simulink model "Figure_2_2_TP_Telecom_modulation_demodulation_ASK2"  (R2020a)
settings: Solver=VariableStepAuto  StartTime=0.0  StopTime=10.0  RelTol=1e-3
libraries: simulink x2, dspsigops x2, dspsrcs4 x2, commrandsrc3 x1, dsparch4 x1, commsink2 x1, commfilt2 x1, commutil2 x1
settings Model: Creator=iba  LastModifiedBy=iba

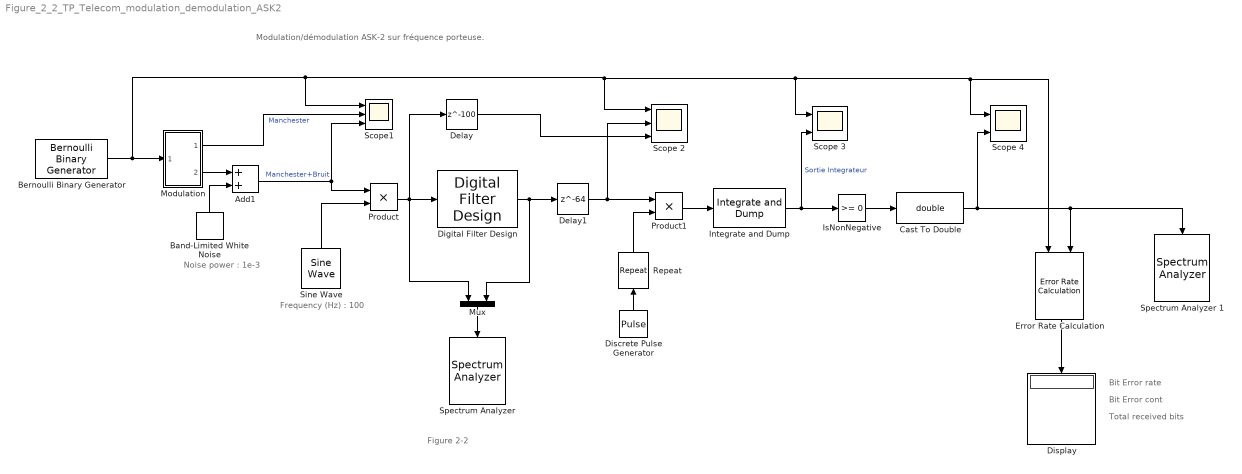
== system Figure_2_2_TP_Telecom_modulation_demodulation_ASK2 ==
  note: Figure 2-2
  note: Noise power : 1e-3
  note: Modulation/démodulation ASK-2 sur fréquence porteuse.
  note: Frequency (Hz) : 100
  note: Bit Error rate
  note: Bit Error cont
  note: Total received bits
  Add1 : Sum
  "Band-Limited White Noise " : simulink/Sources/Band-Limited White Noise  Cov=[1e-3]  Ts=1  seed=[1]
  "Bernoulli Binary Generator " : commrandsrc3/Bernoulli Binary Generator  ProbabilityOfZero=0.5  SeedSource=Parameter  Seed=25.  SampleTime=1  SamplesPerFrame=1  OutputDataType=double  SimulateUsing=Interpreted execution
  Cast To Double : DataTypeConversion  OutDataTypeStr=double
  "Delay " : Delay  DelayLength=100  InitialCondition=0
  "Delay1 " : Delay  DelayLength=64  InitialCondition=0
  "Digital Filter Design " : dsparch4/Digital Filter Design  mwdsp_browser_bugfix_var=off
  Discrete Pulse Generator : DiscretePulseGenerator  Period=10  PulseWidth=4
  "Display " : Display
  Error Rate Calculation : commsink2/Error Rate Calculation  N=1  st_delay=0  cp_mode=Entire frame  subframe=[]  PMode=Port  WsName=ErrorVec  RsMode2=off  stop=off  numErr=100  maxBits=1e6
  Integrate and Dump : commfilt2/Integrate and Dump  obssamples=2  offsetsamples=0  nodump=off  roundingMode=Floor  overflowMode=off
  IsNonNegative : simulink/Logic and Bit Operations/Compare To Zero  relop=>=  OutDataTypeStr=boolean
  Modulation : Subsystem
  Mux : Mux  Inputs=2
  "Product " : Product
  "Product1 " : Product
  Repeat : dspsigops/Repeat  N=50  RateOptions=Allow multirate processing  ic=0  mode=Unused parameter value
  Scope 2 : Scope  NumInputPorts=3
  Scope 3 : Scope  NumInputPorts=2
  Scope 4 : Scope  NumInputPorts=2
  "Scope1 " : Scope  NumInputPorts=3
  Sine Wave : dspsrcs4/Sine Wave  Amplitude=1  Frequency=100  Phase=0  SampleMode=Discrete  OutComplex=Real  CompMethod=Trigonometric fcn  TableSize=Speed  SampleTime=1  SamplesPerFrame=1  ResetState=Restart at time zero  OutputFrames=off  dataType=double  wordLen=16  udDataType=sfix(16)  fracBitsMode=Best precision  numFracBits=15  OutDataTypeStr=double  LastOutDataTypeStr=double
  "Spectrum Analyzer " : SpectrumAnalyzer
  Spectrum Analyzer 1 : SpectrumAnalyzer
  wires:
  "Bernoulli Binary Generator "/1 -> "Scope1 "/1, Error Rate Calculation/1, Scope 4/1, Scope 3/1, Scope 2/1, Modulation/1(IN1)
  Modulation/1(OUT1) -> "Scope1 "/2  "Manchester"
  Modulation/2(OUT2) -> Add1/1
  "Band-Limited White Noise "/1 -> Add1/2
  Add1/1 -> "Scope1 "/3, "Product "/1  "Manchester+Bruit"
  Sine Wave/1 -> "Product "/2
  "Product "/1 -> Mux/1, "Delay "/1, "Digital Filter Design "/1
  "Digital Filter Design "/1 -> "Delay1 "/1, Mux/2
  Mux/1 -> "Spectrum Analyzer "/1
  "Delay1 "/1 -> Scope 2/2, "Product1 "/1
  "Delay "/1 -> Scope 2/3
  "Product1 "/1 -> Integrate and Dump/1
  Repeat/1 -> "Product1 "/2
  Discrete Pulse Generator/1 -> Repeat/1
  Cast To Double/1 -> Scope 4/2, Spectrum Analyzer 1/1, Error Rate Calculation/2
  Integrate and Dump/1 -> Scope 3/2, IsNonNegative/1  "Sortie Integrateur"
  IsNonNegative/1 -> Cast To Double/1
  Error Rate Calculation/1 -> "Display "/1

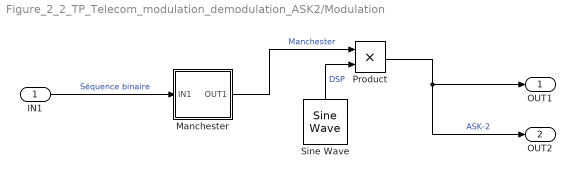
== system Figure_2_2_TP_Telecom_modulation_demodulation_ASK2/Modulation ==
  IN1 : Inport
  Manchester : Subsystem
  "Product " : Product  OutDataTypeStr=double  LockScale=on
  Sine Wave : dspsrcs4/Sine Wave  Amplitude=1  Frequency=5  Phase=0  SampleMode=Discrete  OutComplex=Real  CompMethod=Trigonometric fcn  TableSize=Speed  SampleTime=1  SamplesPerFrame=1  ResetState=Restart at time zero  OutputFrames=off  dataType=Inherit via back propagation  wordLen=16  udDataType=sfix(16)  fracBitsMode=Best precision  numFracBits=15  OutDataTypeStr=Inherit: Inherit via back propagation  LastOutDataTypeStr=Inherit: Inherit via back propagation
  OUT1 : Outport
  OUT2 : Outport  Port=2
  wires:
  "Product "/1 -> OUT2/1, OUT1/1  "ASK-2"
  Sine Wave/1 -> "Product "/2  "DSP"
  Manchester/1(OUT1) -> "Product "/1  "Manchester"
  IN1/1 -> Manchester/1(IN1)  "Séquence binaire"

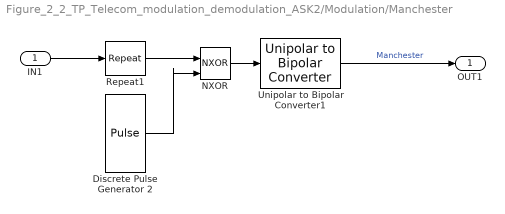
== system Figure_2_2_TP_Telecom_modulation_demodulation_ASK2/Modulation/Manchester ==
  IN1 : Inport
  "Discrete Pulse Generator 2  " : DiscretePulseGenerator  SampleTime=0.01
  "NXOR " : Logic  Operator=NXOR  IconShape=distinctive  AllPortsSameDT=off  OutDataTypeStr=boolean
  Repeat1 : dspsigops/Repeat  N=2  InputProcessing=Columns as channels (frame based)  RateOptions=Enforce single-rate processing  ic=0  mode=Unused parameter value
  Unipolar to Bipolar Converter1 : commutil2/Unipolar to Bipolar Converter  M=2  polarity=Positive  dataType=double
  OUT1 : Outport
  wires:
  IN1/1 -> Repeat1/1
  "NXOR "/1 -> Unipolar to Bipolar Converter1/1
  "Discrete Pulse Generator 2  "/1 -> "NXOR "/2
  Unipolar to Bipolar Converter1/1 -> OUT1/1  "Manchester"
  Repeat1/1 -> "NXOR "/1
